simulink model "Dron_neuron_XY"  (R2019a)
settings: Solver=FixedStepAuto  StartTime=0.0  StopTime=100  FixedStep=1e-4  RelTol=1e-3
values from neighbouring files (symbols this model uses):
  delay = 0.001    [dron.m]
  eta = 20    [dron.m]
  force_max = force_max_1 * 4    (= 47.088)    [dron.m]
  g = 9.81    [dron.m]
  Iunx = 0.1820    (= 0.182)    [dron.m]
  Iunz = 0.2506    [dron.m]
  Ixx = 0.02276    [dron.m]
  Iyy = Ixx    (= 0.02276)    [dron.m]
  Izz = 0.03132    [dron.m]
  k1 = 6    [dron.m]
  k2 = 6    [dron.m]
  k3 = 10    [dron.m]
  k_x = 10    [dron.m]
  k_y = 10    [dron.m]
  k_z = 1    [dron.m]
  m = 1    [dron.m]
  n = 7    [dron.m]
  nn_on = 1    [dron.m]
  torque_max_rp = omega_max ^ 2 * 2 * b * l    (= 5.2974)    [dron.m]
  torque_max_y = omega_max ^ 2 * 2 * d    (= 0.686230416)    [dron.m]
undefined symbols (not defined in the file or in its folder): sigbuilder_block
libraries: simulink_extras x9, neural x4, simulink x2, powerlib_extras x1
(part 2 of 2)

== system Dron_neuron_XY/Motors Control/Backstepping + NN (Roll)/Neural Network ==
  alpha : Inport
  alpha'_e : Inport  Port=2
  alpha' : Inport  Port=3
  Constant1 : Constant  Value=eta*ones(1,n+1)
  Constant2 : Constant  Value=rand(n,1)
  Constant3 : Constant  Value=randn(n,1)
  Gain : Gain  Gain=0.05
  Gain1 : Gain  Gain=0.05
  Integrator : Integrator  InitialCondition=zeros(1, n+1)
  Mux : Mux  Inputs=2
  Product : Product
  Product1 : Product  Inputs=3
  Product2 : Product
  Sum : Sum  Inputs=+
  Sum1 : Sum  Inputs=|++
  tansig : neural/Transfer Functions/tansig
      settings: SourceProductName=MATLAB Runtime - Deep Learning Toolbox  SourceProductBaseCode=Missing
  u : Outport
  weights and bias : Outport  Port=2
  wires:
  alpha/1 -> Product2/1
  tansig/1 -> Mux/1
  alpha'/1 -> Mux/2
  Sum1/1 -> tansig/1
  Mux/1 -> Product1/1, Product/1
  Sum/1 -> u/1
  Integrator/1 -> weights and bias/1, Product/2
  Product/1 -> Sum/1
  Product1/1 -> Integrator/1
  alpha'_e/1 -> Product1/2
  Constant1/1 -> Product1/3
  Constant2/1 -> Gain/1
  Product2/1 -> Sum1/1
  Constant3/1 -> Gain1/1
  Gain/1 -> Product2/2
  Gain1/1 -> Sum1/2

== system Dron_neuron_XY/Motors Control/Backstepping + NN (Roll)/alpha'_d' ==
  alpha_d' : Inport
  alpha_e : Inport  Port=2
  alpha' : Inport  Port=3
  Add : Sum  Inputs=+-
  Constant : Constant  Value=k1
  Derivative1 : Derivative
  Product : Product
  alpha'_d : Sum
  alpha'_d' : Outport
  alpha'_e : Outport  Port=2
  wires:
  Constant/1 -> Product/2
  Add/1 -> alpha'_e/1
  alpha'_d/1 -> Add/1, Derivative1/1
  Product/1 -> alpha'_d/1
  alpha'/1 -> Add/2
  alpha_e/1 -> Product/1
  Derivative1/1 -> alpha'_d'/1
  alpha_d'/1 -> alpha'_d/2

== system Dron_neuron_XY/Motors Control/Backstepping + NN (Yaw)/Control Signal ==
  theta' : Inport
  alpha' : Inport  Port=2
  phi'_e : Inport  Port=3
  phi'_d' : Inport  Port=4
  Add : Sum  Inputs=+-
  Add1 : Sum  Inputs=-++
  Constant : Constant  Value=Iyy
  Constant1 : Constant  Value=Izz
  Constant2 : Constant  Value=k2
  Constant3 : Constant  Value=Ixx
  Product : Product
  Product1 : Product  Inputs=**/
  Product2 : Product
  Product3 : Product
  u : Outport
  wires:
  theta'/1 -> Product/2
  alpha'/1 -> Product/1
  Product/1 -> Product1/1
  Constant3/1 -> Add/1
  Constant/1 -> Add/2
  Add/1 -> Product1/2
  Product1/1 -> Add1/1
  phi'_e/1 -> Product2/1
  Constant2/1 -> Product2/2
  Product2/1 -> Add1/2
  Constant1/1 -> Product3/2, Product1/3
  Add1/1 -> Product3/1
  Product3/1 -> u/1
  phi'_d'/1 -> Add1/3

== system Dron_neuron_XY/Motors Control/Backstepping + NN (Yaw)/Neural Network ==
  phi : Inport
  phi'_e : Inport  Port=2
  phi' : Inport  Port=3
  Constant1 : Constant  Value=eta*ones(1,n+1)
  Constant2 : Constant  Value=rand(n,1)
  Constant3 : Constant  Value=randn(n,1)
  Gain1 : Gain  Gain=0.05
  Gain2 : Gain  Gain=0.05
  Integrator : Integrator  InitialCondition=zeros(1, n+1)
  Mux : Mux  Inputs=2
  Product : Product
  Product1 : Product  Inputs=3
  Product2 : Product
  Sum : Sum  Inputs=+
  Sum1 : Sum  Inputs=|++
  tansig : neural/Transfer Functions/tansig
      settings: SourceProductName=MATLAB Runtime - Deep Learning Toolbox  SourceProductBaseCode=Missing
  u : Outport
  weights and bias : Outport  Port=2
  wires:
  phi/1 -> Product2/1
  tansig/1 -> Mux/1
  phi'/1 -> Mux/2
  Sum1/1 -> tansig/1
  Mux/1 -> Product1/1, Product/1
  Sum/1 -> u/1
  Integrator/1 -> weights and bias/1, Product/2
  Product/1 -> Sum/1
  Product1/1 -> Integrator/1
  phi'_e/1 -> Product1/2
  Constant1/1 -> Product1/3
  Constant2/1 -> Gain2/1
  Product2/1 -> Sum1/1
  Constant3/1 -> Gain1/1
  Gain2/1 -> Product2/2
  Gain1/1 -> Sum1/2

== system Dron_neuron_XY/Motors Control/Backstepping + NN (Yaw)/phi'_d' ==
  phi_d' : Inport
  phi_e : Inport  Port=2
  phi' : Inport  Port=3
  Add : Sum  Inputs=+-
  Constant : Constant  Value=k1
  Derivative1 : Derivative
  Product : Product
  phi'_d : Sum
  phi'_d' : Outport
  phi'_e : Outport  Port=2
  wires:
  Constant/1 -> Product/2
  Add/1 -> phi'_e/1
  phi'_d/1 -> Add/1, Derivative1/1
  Product/1 -> phi'_d/1
  phi'/1 -> Add/2
  phi_e/1 -> Product/1
  Derivative1/1 -> phi'_d'/1
  phi_d'/1 -> phi'_d/2

== system Dron_neuron_XY/Motors Control/Backstepping + NN (Z)/Control Signal ==
  alpha : Inport
  theta : Inport  Port=2
  z'_d' : Inport  Port=3
  z'_e : Inport  Port=4
  z' : Inport  Port=5
  Add : Sum  Inputs=++++
  Constant : Constant  Value=g
  Constant1 : Constant  Value=m
  Cos : Trigonometry  Operator=cos
  Cos1 : Trigonometry  Operator=cos
  Gain1 : Gain  Gain=k_z
  Gain2 : Gain  Gain=k3
  Product : Product
  Product1 : Product  Inputs=**/
  u : Outport
  wires:
  alpha/1 -> Cos/1
  theta/1 -> Cos1/1
  Product/1 -> Product1/3
  Constant1/1 -> Product1/1
  Add/1 -> Product1/2
  Product1/1 -> u/1
  Constant/1 -> Add/1
  z'/1 -> Gain1/1
  Gain1/1 -> Add/2
  z'_d'/1 -> Add/3
  z'_e/1 -> Gain2/1
  Gain2/1 -> Add/4
  Cos/1 -> Product/1
  Cos1/1 -> Product/2

== system Dron_neuron_XY/Motors Control/Backstepping + NN (Z)/Neural Network ==
  z : Inport
  z'_e : Inport  Port=2
  z' : Inport  Port=3
  Constant1 : Constant  Value=eta*ones(1,n+1)
  Constant2 : Constant  Value=rand(n,1)
  Constant3 : Constant  Value=randn(n,1)
  Gain : Gain  Gain=0.5
  Gain1 : Gain  Gain=0.5
  Integrator : Integrator  InitialCondition=zeros(1, n+1)
  Mux : Mux  Inputs=2
  Product : Product
  Product1 : Product  Inputs=3
  Product2 : Product
  Sum : Sum  Inputs=+
  Sum1 : Sum  Inputs=|++
  tansig : neural/Transfer Functions/tansig
      settings: SourceProductName=MATLAB Runtime - Deep Learning Toolbox  SourceProductBaseCode=Missing
  u : Outport
  weights and bias : Outport  Port=2
  wires:
  z/1 -> Product2/1
  tansig/1 -> Mux/1
  z'/1 -> Mux/2
  Sum1/1 -> tansig/1
  Mux/1 -> Product1/1, Product/1
  Sum/1 -> u/1
  Integrator/1 -> weights and bias/1, Product/2
  Product/1 -> Sum/1
  Product1/1 -> Integrator/1
  z'_e/1 -> Product1/2
  Constant1/1 -> Product1/3
  Constant2/1 -> Gain/1
  Product2/1 -> Sum1/1
  Constant3/1 -> Gain1/1
  Gain/1 -> Product2/2
  Gain1/1 -> Sum1/2

== system Dron_neuron_XY/Motors Control/Backstepping + NN (Z)/z'_d' ==
  z_d' : Inport
  z_e : Inport  Port=2
  z' : Inport  Port=3
  Add : Sum  Inputs=+-
  Constant : Constant  Value=k1
  Derivative : Derivative
  Product : Product
  z'_d : Sum
  z'_d' : Outport
  z'_e : Outport  Port=2
  wires:
  z_e/1 -> Product/1
  Constant/1 -> Product/2
  Product/1 -> z'_d/1
  z_d'/1 -> z'_d/2
  z'_d/1 -> Add/1, Derivative/1
  Derivative/1 -> z'_d'/1
  Add/1 -> z'_e/1
  z'/1 -> Add/2

== system Dron_neuron_XY/Subsystem/Linear accelerations1/Body to world - x ==
  alpha : Inport
  theta : Inport  Port=2
  "phi " : Inport  Port=3
  X body acceleration : Inport  Port=4
  Add1 : Sum
  Cos4 : Trigonometry  Operator=cos
  Cos5 : Trigonometry  Operator=cos
  Product : Product
  Product1 : Product  Inputs=3
  Product4 : Product
  Sin3 : Trigonometry
  Sin4 : Trigonometry
  Sin5 : Trigonometry
  converted value : Outport
  wires:
  X body acceleration/1 -> Product/2
  Product/1 -> converted value/1
  Add1/1 -> Product/1
  Sin3/1 -> Product1/3
  Product1/1 -> Add1/2
  Sin4/1 -> Product4/2
  alpha/1 -> Sin5/1, Cos5/1
  "phi "/1 -> Sin4/1, Cos4/1
  Cos5/1 -> Product1/1
  Product4/1 -> Add1/1
  theta/1 -> Sin3/1
  Sin5/1 -> Product4/1
  Cos4/1 -> Product1/2

== system Dron_neuron_XY/Subsystem/Linear accelerations1/Body to world - y ==
  alpha : Inport
  theta : Inport  Port=2
  phi : Inport  Port=3
  Y body acceleration : Inport  Port=4
  Add2 : Sum
  Cos2 : Trigonometry  Operator=cos
  Cos3 : Trigonometry  Operator=cos
  Product : Product
  Product2 : Product  Inputs=3
  Product5 : Product
  Sin : Trigonometry
  Sin1 : Trigonometry
  Sin2 : Trigonometry
  converted value : Outport
  wires:
  Cos2/1 -> Product5/2
  Y body acceleration/1 -> Product/2
  Product/1 -> converted value/1
  alpha/1 -> Sin2/1, Cos3/1
  Add2/1 -> Product/1
  Product2/1 -> Add2/2
  phi/1 -> Cos2/1, Sin1/1
  Cos3/1 -> Product2/1
  Sin1/1 -> Product2/2
  theta/1 -> Sin/1
  Product5/1 -> Add2/1
  Sin/1 -> Product2/3
  Sin2/1 -> Product5/1

== system Dron_neuron_XY/Subsystem/Linear accelerations1/Body to world - z ==
  alpha : Inport
  theta : Inport  Port=2
  Z body acceleration : Inport  Port=3
  Cos : Trigonometry  Operator=cos
  Cos1 : Trigonometry  Operator=cos
  Product : Product  Inputs=3
  converted value : Outport
  wires:
  Z body acceleration/1 -> Product/3
  Product/1 -> converted value/1
  Cos/1 -> Product/1
  Cos1/1 -> Product/2
  alpha/1 -> Cos1/1
  theta/1 -> Cos/1
